simulink model "seesawHost"  (R2013b)
settings: Solver=FixedStepDiscrete  StartTime=0.0  StopTime=Inf  FixedStep=Ts  RelTol=1e-3
InitFcn:
  | mario = w32serial('COM50');
  | princess = w32serial('COM48');
  | Ts = 0.1;
  | 
  | fopen(mario);
  | fopen(princess);
StopFcn:
  | fclose(mario)
  | fclose(princess)
libraries: aerolibanimutils x1
settings Model: Creator=scastro  LastModifiedBy=scastro

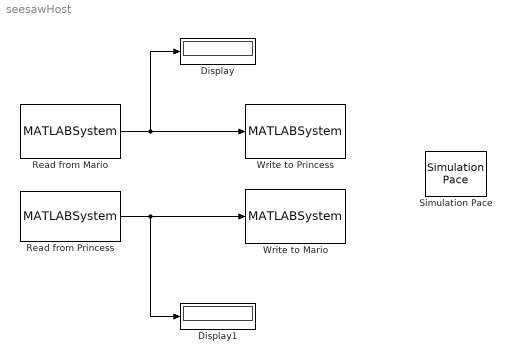
== system seesawHost ==
  Display : Display
  Display1 : Display
  Read from Mario : MATLABSystem  System=w32read  SimulateUsing=Interpreted execution  COMObj=mario  DataType=uint8  DataSize=1  DataLength=1  Mailbox=2
      mask Type: w32read
      mask Display:
      | disp('w32read');
      | port_label('output',1,'msg');
  Read from Princess : MATLABSystem  System=w32read  SimulateUsing=Interpreted execution  COMObj=princess  DataType=uint8  DataSize=1  DataLength=1  Mailbox=3
      mask Type: w32read
      mask Display:
      | disp('w32read');
      | port_label('output',1,'msg');
  Simulation Pace : aerolibanimutils/Simulation Pace  SimulationPace=1  SleepMode=MATLAB Thread  OutputPaceError=off  SampleTime=-1
      settings: AttributesFormatString=%<SimulationPace> sec/sec
  Write to Mario : MATLABSystem  System=w32write  SimulateUsing=Interpreted execution  COMObj=mario  DataType=uint8  DataSize=1  DataLength=1  Mailbox=3
      mask Type: w32write
      mask Display:
      | disp('w32write');
      | port_label('input',1,'data');
  Write to Princess : MATLABSystem  System=w32write  SimulateUsing=Interpreted execution  COMObj=princess  DataType=uint8  DataSize=1  DataLength=1  Mailbox=2
      mask Type: w32write
      mask Display:
      | disp('w32write');
      | port_label('input',1,'data');
  wires:
  Read from Princess/1 -> Write to Mario/1, Display1/1
  Read from Mario/1 -> Display/1, Write to Princess/1
